simulink model "ADIA"  (R2018b)
settings: Solver=FixedStepDiscrete  StartTime=0.0  StopTime=10.0  FixedStep=0.02  RelTol=1e-3
undefined symbols (not defined in the file or in its folder): ACC_State_Active, ACC_State_BrakeOnly, ACC_State_Suspended, ACC_State_WaitingRise, ADAS_AEBBrakingProg, ADAS_DeclControlReq, ADAS_DriveOff, ADAS_ESCHoldReq_NotHold, ADASDecType_ACC, ADASDecType_AEB, ADIA_ACC_Acceleration_OOR_DecCount_C, ADIA_ACC_Acceleration_OOR_Duration_C, ADIA_ACC_Acceleration_OOR_IncCount_C, ADIA_ACC_Acceleration_OOR_LLim_C, ADIA_ACC_Acceleration_OOR_ULim_C, ADIA_ACC_AccelTrqReq_MixedDia_ULim_C, ADIA_ACC_AccelTrqReq_ULim_C, ADIA_ACC_Deceleration_Mixed_ULim_C, ADIA_ACC_Deceleration_OOR_DecCount_C, ADIA_ACC_Deceleration_OOR_Duration_C, ADIA_ACC_Deceleration_OOR_IncCount_C, ADIA_ACC_Deceleration_OOR_LLim_C, ADIA_ACC_Deceleration_OOR_ULim_C, ADIA_ACC_DriveOff_Distance_C, ADIA_ACC_DriveOff_TimeLim_C, ADIA_ACC_ReqMixed_DecCount_C, ADIA_ACC_ReqMixed_Duration_C, ADIA_ACC_ReqMixed_IncCount_C, ADIA_AccPedalRaw_MaxLim_C, ADIA_AccPedalRaw_MinLim_C, ADIA_ADAS_HoldDecReq_Set_C, ADIA_ADAS_HoldRConfirm_TimeLim_C, ADIA_ADAS_HoldVehSpd_Lim_C, ADIA_AEB_VehSpdDec_LLim_C, ADIA_AEB_VehSpdDec_ULim_C, ADIA_ASWFault_OvrdEn_C, ADIA_ASWFault_OvrdValue_C, ADIA_BatteryOutOfRange_DecCount_C, ADIA_BatteryOutOfRange_Duration_C, ADIA_BatteryOutOfRange_IncCount_C, ADIA_BattVolt_MaxLim_C, ADIA_BattVolt_MinLim_C, ADIA_BCM3_33C_InvBrkLight_DecCount_C, ADIA_BCM3_33C_InvBrkLight_Duration_C, ADIA_BCM3_33C_InvBrkLight_IncCount_C, ADIA_BCM_BattVolt_OvrdEn_C, ADIA_BCM_BattVolt_OvrdVal_C, ADIA_BCM_BrakeLampStaus_OvrdEn_C, ADIA_BCM_BrakeLampStaus_OvrdVal_C, ADIA_BCM_CHMSLStaus_OvrdEn_C, ADIA_BCM_CHMSLStaus_OvrdVal_C, ADIA_BCM_LeftTurnSwSt_OvrdEn_C, ADIA_BCM_LeftTurnSwSt_OvrdVal_C, ADIA_BCM_RightTurnSwSt_OvrdEn_C, ADIA_BCM_RightTurnSwSt_OvrdVal_C, ADIA_BCM_TurnSwFailure_DecCount_C, ADIA_BCM_TurnSwFailure_Duration_C, ADIA_BCM_TurnSwFailure_IncCount_C, ADIA_BSWFault_Ignore_C, ADIA_BSWFault_OvrdEn_C ... (+281)
libraries: simulink x208
(part 1 of 10)
settings Model: Creator=ZWG  LastModifiedBy=xiaoyang
settings OptimizationCC: DefaultParameterBehavior=Inlined  EnhancedBackFolding=on  PassReuseOutputArgsAs=Individual arguments  ZeroExternalMemoryAtStartup=off  ZeroInternalMemoryAtStartup=off  OptimizeBlockOrder=speed  DifferentSizesBufferReuse=on  OptimizationCustomize=off
settings DebuggingCC: ParameterTunabilityLossMsg=error
settings SFSimCC: MATLABDynamicMemAlloc=off
settings RTWCC: SystemTargetFile=autosar.tlc  GenCodeOnly=on  TemplateMakefile=ert_default_tmf  Description=AUTOSAR  GenerateReport=on  IncludeHyperlinkInReport=on  LaunchReport=on  GenerateTraceInfo=on  GenerateTraceReport=on  GenerateTraceReportSl=on  GenerateTraceReportSf=on  GenerateTraceReportEml=on
settings CodeAppCC: ForceParamTrailComments=on  IgnoreCustomStorageClasses=off  OperatorAnnotations=on  SimulinkDataObjDesc=on  SFDataObjDesc=on  InsertBlockDesc=on
settings STFCustomTargetCC: TargetLangStandard=C99 (ISO)  MultiwordLength=256  ParMdlRefBuildCompliant=on  CompOptLevelCompliant=on  IncludeMdlTerminateFcn=off  CombineOutputUpdateFcns=on  SuppressErrorStatus=on  ERTCustomFileBanners=on  SupportNonFinite=off  SupportComplex=off  SupportContinuousTime=off  SupportNonInlinedSFcns=off  RemoveResetFunc=on  MATLABClassNameForMDSCustomization=Simulink.SoftwareTarget.ERTCustomization  AutosarCompliant=on  UseToolchainInfoCompliant=on  LookupTableObjectStructAxisOrder=2,1,3,4,...  LUTObjectStructOrderEvenSpacing=Size,Table,Breakpoints  SystemTargetFile=autosar.tlc
settings ERTTargetCC: TargetLangStandard=C99 (ISO)  ConcurrentExecutionCompliant=off  IncludeMdlTerminateFcn=off  SuppressErrorStatus=on  SupportNonFinite=off  SupportComplex=off  ModelStepFunctionPrototypeControlCompliant=off  CPPClassGenCompliant=off  AutosarCompliant=on  LookupTableObjectStructAxisOrder=2,1,3,4,...  LUTObjectStructOrderEvenSpacing=Size,Table,Breakpoints  GenerateASAP2=on  InlinedParameterPlacement=NonHierarchical  ERTCustomFileTemplate=example_file_process.tlc

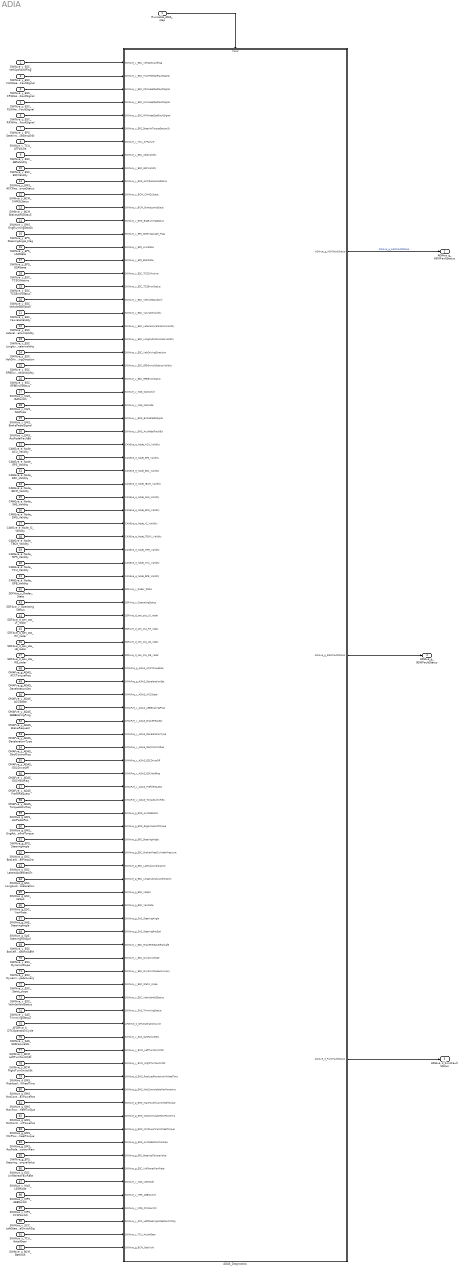
== system ADIA ==
  Runnable_ADIA_step : Inport  SampleTime=0.02  OutputFunctionCall=on
  SWINve_y_ESC_VehSpdValidFlag : Inport  Port=2  OutDataTypeStr=uint8
  SWINve_y_ESC_FLWHeelSpdFaultSignal : Inport  Port=3  OutDataTypeStr=uint8
  SWINve_y_ESC_FRWHeelSpdFaultSignal : Inport  Port=4  OutDataTypeStr=uint8
  SWINve_y_ESC_RLWHeelSpdFaultSignal : Inport  Port=5  OutDataTypeStr=uint8
  SWINve_y_ESC_RRWHeelSpdFaultSignal : Inport  Port=6  OutDataTypeStr=uint8
  SWINve_y_EPS_SteerintTorqueSensorSt : Inport  Port=7  OutDataTypeStr=uint8
  SWINve_y_TCU_ATFailure : Inport  Port=8  OutDataTypeStr=uint8
  SWINve_y_ESC_ABSValidity : Inport  Port=9  OutDataTypeStr=uint8
  SWINve_y_ESC_ESCValidity : Inport  Port=10  OutDataTypeStr=uint8
  SWINve_y_EMS_ACCResponseStatus : Inport  Port=11  OutDataTypeStr=uint8
  SWINve_y_BCM_CHMSLStaus : Inport  Port=12  OutDataTypeStr=uint8
  SWINve_y_BCM_BrakeLampStaus : Inport  Port=13  OutDataTypeStr=uint8
  SWINve_y_EMS_EngRunningStatus : Inport  Port=14  OutDataTypeStr=uint8
  SWINve_y_EPS_SteeringAngle_Flag : Inport  Port=15  OutDataTypeStr=uint8
  SWINve_y_EPS_LKAState : Inport  Port=16  OutDataTypeStr=uint8
  SWINve_y_EPS_ESAState : Inport  Port=17  OutDataTypeStr=uint8
  SWINve_y_ESC_TCSCtlActive : Inport  Port=18  OutDataTypeStr=uint8
  SWINve_y_ESC_TCSErrorStatus : Inport  Port=19  OutDataTypeStr=uint8
  SWINve_y_ESC_VehicleStandstill : Inport  Port=20  OutDataTypeStr=uint8
  SWINve_y_ESC_YawrateValidity : Inport  Port=21  OutDataTypeStr=uint8
  SWINve_y_ESC_LateralAccelarationValidity : Inport  Port=22  OutDataTypeStr=uint8
  SWINve_y_ESC_LongitudinalAccelervalidity : Inport  Port=23  OutDataTypeStr=uint8
  SWINve_y_ESC_VehDrivingDirection : Inport  Port=24  OutDataTypeStr=uint8
  SWINve_y_ESC_EPBSwitchStaticsValidity : Inport  Port=25  OutDataTypeStr=uint8
  SWINve_y_ESC_EPBErrorStatus : Inport  Port=26  OutDataTypeStr=uint8
  SWINve_y_Mp5_ISASwitch : Inport  Port=27  OutDataTypeStr=uint8
  SWINve_y_Mp5_ISAMode : Inport  Port=28  OutDataTypeStr=uint8
  SWINve_y_EMS_BrakePedalSignal : Inport  Port=29  OutDataTypeStr=uint8
  SWINve_y_EMS_AccPedalFaultBit : Inport  Port=30  OutDataTypeStr=uint8
  CANEve_e_Node_ACU_Validity : Inport  Port=31  OutDataTypeStr=Enum: SPARte_e_Validity  PortDimensions=1
  CANEve_e_Node_EPS_Validity : Inport  Port=32  OutDataTypeStr=Enum: SPARte_e_Validity  PortDimensions=1
  CANEve_e_Node_ESC_Validity : Inport  Port=33  OutDataTypeStr=Enum: SPARte_e_Validity  PortDimensions=1
  CANEve_e_Node_IBCM_Validity : Inport  Port=34  OutDataTypeStr=Enum: SPARte_e_Validity  PortDimensions=1
  CANEve_e_Node_SAS_Validity : Inport  Port=35  OutDataTypeStr=Enum: SPARte_e_Validity  PortDimensions=1
  CANEve_e_Node_EMS_Validity : Inport  Port=36  OutDataTypeStr=Enum: SPARte_e_Validity  PortDimensions=1
  CANEve_e_Node_IC_Validity : Inport  Port=37  OutDataTypeStr=Enum: SPARte_e_Validity  PortDimensions=1
  CANEve_e_Node_TBOX_Validity : Inport  Port=38  OutDataTypeStr=Enum: SPARte_e_Validity  PortDimensions=1
  CANEve_e_Node_MP5_Validity : Inport  Port=39  OutDataTypeStr=Enum: SPARte_e_Validity  PortDimensions=1
  CANEve_e_Node_TCU_Validity : Inport  Port=40  OutDataTypeStr=Enum: SPARte_e_Validity  PortDimensions=1
  CANEve_e_Node_EPB_Validity : Inport  Port=41  OutDataTypeStr=Enum: SPARte_e_Validity  PortDimensions=1
  SDFAve_y_Radar_State : Inport  Port=42  OutDataTypeStr=UInt8
  SDFAve_y_OperatingStatus : Inport  Port=43  OutDataTypeStr=UInt8
  SDFAve_d_sen_sta_LF_radar : Inport  Port=44  OutDataTypeStr=UInt16
  SDFAve_d_sen_sta_RF_radar : Inport  Port=45  OutDataTypeStr=UInt16
  SDFAve_d_sen_sta_LB_radar : Inport  Port=46  OutDataTypeStr=UInt16
  SDFAve_d_sen_sta_RB_radar : Inport  Port=47  OutDataTypeStr=UInt16
  OMAPve_g_ADAS_ACCTorqueReq : Inport  Port=48  OutDataTypeStr=T_M_Nm_Float32  PortDimensions=1
  OMAPve_g_ADAS_DecelerationSet : Inport  Port=49  OutDataTypeStr=T_M_Nm_Float32  PortDimensions=1
  OMAPve_y_ADAS_ACCState : Inport  Port=50  OutDataTypeStr=UInt8  PortDimensions=1
  OMAPve_y_ADAS_AEBBrakingProg : Inport  Port=51  OutDataTypeStr=UInt8  PortDimensions=1
  OMAPve_y_ADAS_BrakeRequest : Inport  Port=52  OutDataTypeStr=UInt8  PortDimensions=1
  OMAPve_y_ADAS_DecelerationType : Inport  Port=53  OutDataTypeStr=UInt8  PortDimensions=1
  OMAPve_y_ADAS_DeclControlReq : Inport  Port=54  OutDataTypeStr=UInt8  PortDimensions=1
  OMAPve_y_ADAS_ESCDriveOff : Inport  Port=55  OutDataTypeStr=UInt8  PortDimensions=1
  OMAPve_y_ADAS_ESCHoldReq : Inport  Port=56  OutDataTypeStr=UInt8  PortDimensions=1
  OMAPve_y_ADAS_PrefillRequest : Inport  Port=57  OutDataTypeStr=UInt8  PortDimensions=1
  OMAPve_y_ADAS_TorqueActivReq : Inport  Port=58  OutDataTypeStr=UInt8  PortDimensions=1
  SWINve_g_EMS_AccPedalPos : Inport  Port=59  OutDataTypeStr=single  PortDimensions=1
  SWINve_g_EMS_EngActualIndTorque : Inport  Port=60  OutDataTypeStr=single  PortDimensions=1
  SWINve_g_EPS_SteeringAngle : Inport  Port=61  OutDataTypeStr=single  PortDimensions=1
  SWINve_g_ESC_BrakeWheelCylinderPressure : Inport  Port=62  OutDataTypeStr=single  PortDimensions=1
  SWINve_g_ESC_LateralAccelaration : Inport  Port=63  OutDataTypeStr=single  PortDimensions=1
  SWINve_g_ESC_LongitudinalAcceleration : Inport  Port=64  OutDataTypeStr=single  PortDimensions=1
  SWINve_g_ESC_VeSpd : Inport  Port=65  OutDataTypeStr=single  PortDimensions=1
  SWINve_g_ESC_YawRate : Inport  Port=66  OutDataTypeStr=single  PortDimensions=1
  SWINve_g_SAS_SteeringAngle : Inport  Port=67  OutDataTypeStr=T_M_Nm_Float32  PortDimensions=1
  SWINve_g_SAS_SteeringRotSpd : Inport  Port=68  OutDataTypeStr=single  PortDimensions=1
  SWINve_y_ESC_BrakeReleasedFailsafe : Inport  Port=69  OutDataTypeStr=uint8  PortDimensions=1
  SWINve_y_ESC_DynamicSlope : Inport  Port=70  OutDataTypeStr=int8  PortDimensions=1
  SWINve_y_ESC_DynamicSlopeAccuracy : Inport  Port=71  OutDataTypeStr=uint8  PortDimensions=1
  SWINve_y_ESC_Static_slope : Inport  Port=72  OutDataTypeStr=int8  PortDimensions=1
  SWINve_y_ESC_VehicleHoldStatus : Inport  Port=73  OutDataTypeStr=uint8  PortDimensions=1
  SWINve_y_SAS_TrimmingStatus : Inport  Port=74  OutDataTypeStr=uint8  PortDimensions=1
  AFDMve_b_DTCOperationCycle : Inport  Port=75  OutDataTypeStr=T_BOOLEAN  PortDimensions=1
  SWINve_y_SAS_SASFailureSts : Inport  Port=76  OutDataTypeStr=uint8
  SWINve_y_BCM_LeftTurnSwitchSt : Inport  Port=77  OutDataTypeStr=uint8
  SWINve_y_BCM_RightTurnSwitchSt : Inport  Port=78  OutDataTypeStr=uint8
  SWINve_d_EMS_RealizedPowertrainWheelTorq : Inport  Port=79  OutDataTypeStr=int16
  SWINve_g_EMS_NotControlableMaxPowertra : Inport  Port=80  OutDataTypeStr=single
  SWINve_g_EMS_MaxPowertrainWheelTorque : Inport  Port=81  OutDataTypeStr=single
  SWINve_g_EMS_NotControlableMinPowertra : Inport  Port=82  OutDataTypeStr=single
  SWINve_g_EMS_MinPowertrainWheelTorque : Inport  Port=83  OutDataTypeStr=single
  SWINve_g_EMS_AccPedalPositionRaw : Inport  Port=84  OutDataTypeStr=single
  SWINve_g_EPS_SteeringTorqueValue : Inport  Port=85  OutDataTypeStr=single
  SWINve_g_ESC_UnfilteredYawRate : Inport  Port=86  OutDataTypeStr=single  PortDimensions=1
  SWINve_y_Mp5_LSSMode : Inport  Port=87  OutDataTypeStr=uint8  PortDimensions=1
  SWINve_y_MP5_AEBSwitch : Inport  Port=88  OutDataTypeStr=uint8  PortDimensions=1
  SWINve_y_MP5_FCWSwitch : Inport  Port=89  OutDataTypeStr=uint8  PortDimensions=1
  SWINve_y_SCC_LeftSteeringWheelSwitchSig : Inport  Port=90  OutDataTypeStr=uint8  PortDimensions=1
  SWINve_y_TCU_ActialGear : Inport  Port=91  OutDataTypeStr=uint8  PortDimensions=1
  SWINve_g_BCM_BattVolt : Inport  Port=92  OutDataTypeStr=single  PortDimensions=1
  ADAS_Diagnostics : Subsystem
  ADIAve_g_ASWFaultStatus : Outport  OutDataTypeStr=UInt32
  ADIAve_g_BSWFaultStatus : Outport  Port=2  OutDataTypeStr=UInt32
  ADIAve_d_FuncFaultStatus : Outport  Port=3  OutDataTypeStr=uint16
  wires:
  SDFAve_d_sen_sta_RB_radar/1 -> ADAS_Diagnostics/46(SDFAve_d_sen_sta_RB_radar)
  SWINve_y_ESC_RRWHeelSpdFaultSignal/1 -> ADAS_Diagnostics/5(SWINve_y_ESC_RRWHeelSpdFaultSignal)
  SDFAve_d_sen_sta_LB_radar/1 -> ADAS_Diagnostics/45(SDFAve_d_sen_sta_LB_radar)
  SDFAve_d_sen_sta_RF_radar/1 -> ADAS_Diagnostics/44(SDFAve_d_sen_sta_RF_radar)
  SWINve_y_EMS_EngRunningStatus/1 -> ADAS_Diagnostics/13(SWINve_y_EMS_EngRunningStatus)
  CANEve_e_Node_IBCM_Validity/1 -> ADAS_Diagnostics/33(CANEve_e_Node_IBCM_Validity)
  SDFAve_d_sen_sta_LF_radar/1 -> ADAS_Diagnostics/43(SDFAve_d_sen_sta_LF_radar)
  SDFAve_y_OperatingStatus/1 -> ADAS_Diagnostics/42(SDFAve_y_OperatingStatus)
  SWINve_y_ESC_ABSValidity/1 -> ADAS_Diagnostics/8(SWINve_y_ESC_ABSValidity)
  CANEve_e_Node_MP5_Validity/1 -> ADAS_Diagnostics/38(CANEve_e_Node_MP5_Validity)
  SWINve_y_BCM_CHMSLStaus/1 -> ADAS_Diagnostics/11(SWINve_y_BCM_CHMSLStaus)
  SDFAve_y_Radar_State/1 -> ADAS_Diagnostics/41(SDFAve_y_Radar_State)
  CANEve_e_Node_ESC_Validity/1 -> ADAS_Diagnostics/32(CANEve_e_Node_ESC_Validity)
  CANEve_e_Node_TBOX_Validity/1 -> ADAS_Diagnostics/37(CANEve_e_Node_TBOX_Validity)
  SWINve_y_EPS_SteerintTorqueSensorSt/1 -> ADAS_Diagnostics/6(SWINve_y_EPS_SteerintTorqueSensorSt)
  SWINve_y_ESC_LongitudinalAccelervalidity/1 -> ADAS_Diagnostics/22(SWINve_y_ESC_LongitudinalAccelervalidity)
  CANEve_e_Node_ACU_Validity/1 -> ADAS_Diagnostics/30(CANEve_e_Node_ACU_Validity)
  SWINve_y_ESC_RLWHeelSpdFaultSignal/1 -> ADAS_Diagnostics/4(SWINve_y_ESC_RLWHeelSpdFaultSignal)
  CANEve_e_Node_EMS_Validity/1 -> ADAS_Diagnostics/35(CANEve_e_Node_EMS_Validity)
  CANEve_e_Node_EPS_Validity/1 -> ADAS_Diagnostics/31(CANEve_e_Node_EPS_Validity)
  CANEve_e_Node_IC_Validity/1 -> ADAS_Diagnostics/36(CANEve_e_Node_IC_Validity)
  SWINve_y_ESC_YawrateValidity/1 -> ADAS_Diagnostics/20(SWINve_y_ESC_YawrateValidity)
  SWINve_y_Mp5_ISASwitch/1 -> ADAS_Diagnostics/26(SWINve_y_Mp5_ISASwitch)
  SWINve_y_ESC_EPBSwitchStaticsValidity/1 -> ADAS_Diagnostics/24(SWINve_y_ESC_EPBSwitchStaticsValidity)
  SWINve_y_EPS_ESAState/1 -> ADAS_Diagnostics/16(SWINve_y_EPS_ESAState)
  CANEve_e_Node_SAS_Validity/1 -> ADAS_Diagnostics/34(CANEve_e_Node_SAS_Validity)
  SWINve_y_BCM_BrakeLampStaus/1 -> ADAS_Diagnostics/12(SWINve_y_BCM_BrakeLampStaus)
  Runnable_ADIA_step/1 -> ADAS_Diagnostics/Trigger
  SWINve_y_EMS_ACCResponseStatus/1 -> ADAS_Diagnostics/10(SWINve_y_EMS_ACCResponseStatus)
  SWINve_y_ESC_EPBErrorStatus/1 -> ADAS_Diagnostics/25(SWINve_y_ESC_EPBErrorStatus)
  SWINve_y_EPS_SteeringAngle_Flag/1 -> ADAS_Diagnostics/14(SWINve_y_EPS_SteeringAngle_Flag)
  SWINve_y_ESC_FRWHeelSpdFaultSignal/1 -> ADAS_Diagnostics/3(SWINve_y_ESC_FRWHeelSpdFaultSignal)
  ADAS_Diagnostics/2(ADIAve_g_BSWFaultStatus) -> ADIAve_g_BSWFaultStatus/1
  SWINve_y_ESC_ESCValidity/1 -> ADAS_Diagnostics/9(SWINve_y_ESC_ESCValidity)
  SWINve_y_TCU_ATFailure/1 -> ADAS_Diagnostics/7(SWINve_y_TCU_ATFailure)
  SWINve_y_ESC_FLWHeelSpdFaultSignal/1 -> ADAS_Diagnostics/2(SWINve_y_ESC_FLWHeelSpdFaultSignal)
  SWINve_y_EPS_LKAState/1 -> ADAS_Diagnostics/15(SWINve_y_EPS_LKAState)
  ADAS_Diagnostics/1(ADIAve_g_ASWFaultStatus) -> ADIAve_g_ASWFaultStatus/1  "ADIAve_g_ASWFaultStatus"
  AFDMve_b_DTCOperationCycle/1 -> ADAS_Diagnostics/74(AFDMve_b_DTCOperationCycle)
  SWINve_y_ESC_VehicleStandstill/1 -> ADAS_Diagnostics/19(SWINve_y_ESC_VehicleStandstill)
  CANEve_e_Node_TCU_Validity/1 -> ADAS_Diagnostics/39(CANEve_e_Node_TCU_Validity)
  CANEve_e_Node_EPB_Validity/1 -> ADAS_Diagnostics/40(CANEve_e_Node_EPB_Validity)
  SWINve_y_ESC_LateralAccelarationValidity/1 -> ADAS_Diagnostics/21(SWINve_y_ESC_LateralAccelarationValidity)
  SWINve_y_ESC_TCSCtlActive/1 -> ADAS_Diagnostics/17(SWINve_y_ESC_TCSCtlActive)
  SWINve_y_EMS_AccPedalFaultBit/1 -> ADAS_Diagnostics/29(SWINve_y_EMS_AccPedalFaultBit)
  SWINve_y_ESC_TCSErrorStatus/1 -> ADAS_Diagnostics/18(SWINve_y_ESC_TCSErrorStatus)
  SWINve_y_ESC_VehDrivingDirection/1 -> ADAS_Diagnostics/23(SWINve_y_ESC_VehDrivingDirection)
  SWINve_y_ESC_VehSpdValidFlag/1 -> ADAS_Diagnostics/1(SWINve_y_ESC_VehSpdValidFlag)
  SWINve_y_Mp5_ISAMode/1 -> ADAS_Diagnostics/27(SWINve_y_Mp5_ISAMode)
  SWINve_y_EMS_BrakePedalSignal/1 -> ADAS_Diagnostics/28(SWINve_y_EMS_BrakePedalSignal)
  SWINve_y_SAS_TrimmingStatus/1 -> ADAS_Diagnostics/73(SWINve_y_SAS_TrimmingStatus)
  SWINve_y_ESC_VehicleHoldStatus/1 -> ADAS_Diagnostics/72(SWINve_y_ESC_VehicleHoldStatus)
  SWINve_y_ESC_Static_slope/1 -> ADAS_Diagnostics/71(SWINve_y_ESC_Static_slope)
  SWINve_y_ESC_DynamicSlopeAccuracy/1 -> ADAS_Diagnostics/70(SWINve_y_ESC_DynamicSlopeAccuracy)
  SWINve_y_ESC_DynamicSlope/1 -> ADAS_Diagnostics/69(SWINve_y_ESC_DynamicSlope)
  SWINve_y_ESC_BrakeReleasedFailsafe/1 -> ADAS_Diagnostics/68(SWINve_y_ESC_BrakeReleasedFailsafe)
  SWINve_g_SAS_SteeringRotSpd/1 -> ADAS_Diagnostics/67(SWINve_g_SAS_SteeringRotSpd)
  SWINve_g_SAS_SteeringAngle/1 -> ADAS_Diagnostics/66(SWINve_g_SAS_SteeringAngle)
  SWINve_g_ESC_YawRate/1 -> ADAS_Diagnostics/65(SWINve_g_ESC_YawRate)
  SWINve_g_ESC_VeSpd/1 -> ADAS_Diagnostics/64(SWINve_g_ESC_VeSpd)
  SWINve_g_ESC_LongitudinalAcceleration/1 -> ADAS_Diagnostics/63(SWINve_g_ESC_LongitudinalAcceleration)
  SWINve_g_ESC_LateralAccelaration/1 -> ADAS_Diagnostics/62(SWINve_g_ESC_LateralAccelaration)
  SWINve_g_ESC_BrakeWheelCylinderPressure/1 -> ADAS_Diagnostics/61(SWINve_g_ESC_BrakeWheelCylinderPressure)
  SWINve_g_EPS_SteeringAngle/1 -> ADAS_Diagnostics/60(SWINve_g_EPS_SteeringAngle)
  SWINve_g_EMS_EngActualIndTorque/1 -> ADAS_Diagnostics/59(SWINve_g_EMS_EngActualIndTorque)
  SWINve_g_EMS_AccPedalPos/1 -> ADAS_Diagnostics/58(SWINve_g_EMS_AccPedalPos)
  OMAPve_y_ADAS_TorqueActivReq/1 -> ADAS_Diagnostics/57(OMAPve_y_ADAS_TorqueActivReq)
  OMAPve_y_ADAS_PrefillRequest/1 -> ADAS_Diagnostics/56(OMAPve_y_ADAS_PrefillRequest)
  OMAPve_y_ADAS_ESCHoldReq/1 -> ADAS_Diagnostics/55(OMAPve_y_ADAS_ESCHoldReq)
  OMAPve_y_ADAS_ESCDriveOff/1 -> ADAS_Diagnostics/54(OMAPve_y_ADAS_ESCDriveOff)
  OMAPve_y_ADAS_DeclControlReq/1 -> ADAS_Diagnostics/53(OMAPve_y_ADAS_DeclControlReq)
  OMAPve_y_ADAS_DecelerationType/1 -> ADAS_Diagnostics/52(OMAPve_y_ADAS_DecelerationType)
  OMAPve_y_ADAS_BrakeRequest/1 -> ADAS_Diagnostics/51(OMAPve_y_ADAS_BrakeRequest)
  OMAPve_y_ADAS_AEBBrakingProg/1 -> ADAS_Diagnostics/50(OMAPve_y_ADAS_AEBBrakingProg)
  OMAPve_y_ADAS_ACCState/1 -> ADAS_Diagnostics/49(OMAPve_y_ADAS_ACCState)
  OMAPve_g_ADAS_DecelerationSet/1 -> ADAS_Diagnostics/48(OMAPve_g_ADAS_DecelerationSet)
  OMAPve_g_ADAS_ACCTorqueReq/1 -> ADAS_Diagnostics/47(OMAPve_g_ADAS_ACCTorqueReq)
  SWINve_y_SAS_SASFailureSts/1 -> ADAS_Diagnostics/75(SWINve_y_SAS_SASFailureSts)
  SWINve_y_BCM_LeftTurnSwitchSt/1 -> ADAS_Diagnostics/76(SWINve_y_BCM_LeftTurnSwitchSt)
  SWINve_y_BCM_RightTurnSwitchSt/1 -> ADAS_Diagnostics/77(SWINve_y_BCM_RightTurnSwitchSt)
  SWINve_d_EMS_RealizedPowertrainWheelTorq/1 -> ADAS_Diagnostics/78(SWINve_d_EMS_RealizedPowertrainWheelTorq)
  SWINve_g_EMS_NotControlableMaxPowertra/1 -> ADAS_Diagnostics/79(SWINve_g_EMS_NotControlableMaxPowertra)
  SWINve_g_EMS_MaxPowertrainWheelTorque/1 -> ADAS_Diagnostics/80(SWINve_g_EMS_MaxPowertrainWheelTorque)
  SWINve_g_EMS_NotControlableMinPowertra/1 -> ADAS_Diagnostics/81(SWINve_g_EMS_NotControlableMinPowertra)
  SWINve_g_EMS_MinPowertrainWheelTorque/1 -> ADAS_Diagnostics/82(SWINve_g_EMS_MinPowertrainWheelTorque)
  SWINve_g_EMS_AccPedalPositionRaw/1 -> ADAS_Diagnostics/83(SWINve_g_EMS_AccPedalPositionRaw)
  SWINve_g_EPS_SteeringTorqueValue/1 -> ADAS_Diagnostics/84(SWINve_g_EPS_SteeringTorqueValue)
  SWINve_g_ESC_UnfilteredYawRate/1 -> ADAS_Diagnostics/85(SWINve_g_ESC_UnfilteredYawRate)
  SWINve_y_MP5_AEBSwitch/1 -> ADAS_Diagnostics/87(SWINve_y_MP5_AEBSwitch)
  SWINve_y_Mp5_LSSMode/1 -> ADAS_Diagnostics/86(SWINve_y_Mp5_LSSMode)
  SWINve_y_MP5_FCWSwitch/1 -> ADAS_Diagnostics/88(SWINve_y_MP5_FCWSwitch)
  SWINve_y_TCU_ActialGear/1 -> ADAS_Diagnostics/90(SWINve_y_TCU_ActialGear)
  SWINve_y_SCC_LeftSteeringWheelSwitchSig/1 -> ADAS_Diagnostics/89(SWINve_y_SCC_LeftSteeringWheelSwitchSig)
  SWINve_g_BCM_BattVolt/1 -> ADAS_Diagnostics/91(SWINve_g_BCM_BattVolt)
  ADAS_Diagnostics/3(ADIAve_d_FuncFaultStatus) -> ADIAve_d_FuncFaultStatus/1

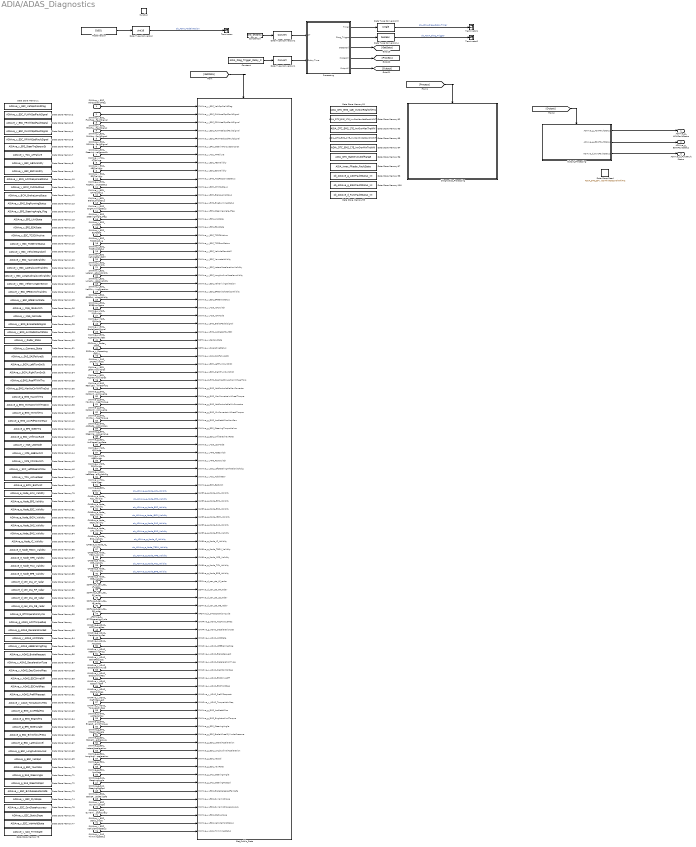
== system ADIA/ADAS_Diagnostics ==
  SWINve_y_ESC_VehSpdValidFlag : Inport
  SWINve_y_ESC_FLWHeelSpdFaultSignal : Inport  Port=2
  SWINve_y_ESC_FRWHeelSpdFaultSignal : Inport  Port=3
  SWINve_y_ESC_RLWHeelSpdFaultSignal : Inport  Port=4
  SWINve_y_ESC_RRWHeelSpdFaultSignal : Inport  Port=5
  SWINve_y_EPS_SteerintTorqueSensorSt : Inport  Port=6
  SWINve_y_TCU_ATFailure : Inport  Port=7
  SWINve_y_ESC_ABSValidity : Inport  Port=8
  SWINve_y_ESC_ESCValidity : Inport  Port=9
  SWINve_y_EMS_ACCResponseStatus : Inport  Port=10
  SWINve_y_BCM_CHMSLStaus : Inport  Port=11
  SWINve_y_BCM_BrakeLampStaus : Inport  Port=12
  SWINve_y_EMS_EngRunningStatus : Inport  Port=13
  SWINve_y_EPS_SteeringAngle_Flag : Inport  Port=14
  SWINve_y_EPS_LKAState : Inport  Port=15
  SWINve_y_EPS_ESAState : Inport  Port=16
  SWINve_y_ESC_TCSCtlActive : Inport  Port=17
  SWINve_y_ESC_TCSErrorStatus : Inport  Port=18
  SWINve_y_ESC_VehicleStandstill : Inport  Port=19
  SWINve_y_ESC_YawrateValidity : Inport  Port=20
  SWINve_y_ESC_LateralAccelarationValidity : Inport  Port=21
  SWINve_y_ESC_LongitudinalAccelervalidity : Inport  Port=22
  SWINve_y_ESC_VehDrivingDirection : Inport  Port=23
  SWINve_y_ESC_EPBSwitchStaticsValidity : Inport  Port=24
  SWINve_y_ESC_EPBErrorStatus : Inport  Port=25
  SWINve_y_Mp5_ISASwitch : Inport  Port=26
  SWINve_y_Mp5_ISAMode : Inport  Port=27
  SWINve_y_EMS_BrakePedalSignal : Inport  Port=28
  SWINve_y_EMS_AccPedalFaultBit : Inport  Port=29
  CANEve_e_Node_ACU_Validity : Inport  Port=30  PortDimensions=1
  CANEve_e_Node_EPS_Validity : Inport  Port=31  PortDimensions=1
  CANEve_e_Node_ESC_Validity : Inport  Port=32  PortDimensions=1
  CANEve_e_Node_IBCM_Validity : Inport  Port=33  PortDimensions=1
  CANEve_e_Node_SAS_Validity : Inport  Port=34  PortDimensions=1
  CANEve_e_Node_EMS_Validity : Inport  Port=35  PortDimensions=1
  CANEve_e_Node_IC_Validity : Inport  Port=36  PortDimensions=1
  CANEve_e_Node_TBOX_Validity : Inport  Port=37  PortDimensions=1
  CANEve_e_Node_MP5_Validity : Inport  Port=38  PortDimensions=1
  CANEve_e_Node_TCU_Validity : Inport  Port=39  PortDimensions=1
  CANEve_e_Node_EPB_Validity : Inport  Port=40  PortDimensions=1
  SDFAve_y_Radar_State : Inport  Port=41
  SDFAve_y_OperatingStatus : Inport  Port=42
  SDFAve_d_sen_sta_LF_radar : Inport  Port=43
  SDFAve_d_sen_sta_RF_radar : Inport  Port=44
  SDFAve_d_sen_sta_LB_radar : Inport  Port=45
  SDFAve_d_sen_sta_RB_radar : Inport  Port=46
  OMAPve_g_ADAS_ACCTorqueReq : Inport  Port=47  OutDataTypeStr=T_M_Nm_Float32  PortDimensions=1
  OMAPve_g_ADAS_DecelerationSet : Inport  Port=48  OutDataTypeStr=T_M_Nm_Float32  PortDimensions=1
  OMAPve_y_ADAS_ACCState : Inport  Port=49  OutDataTypeStr=UInt8  PortDimensions=1
  OMAPve_y_ADAS_AEBBrakingProg : Inport  Port=50  OutDataTypeStr=UInt8  PortDimensions=1
  OMAPve_y_ADAS_BrakeRequest : Inport  Port=51  OutDataTypeStr=UInt8  PortDimensions=1
  OMAPve_y_ADAS_DecelerationType : Inport  Port=52  OutDataTypeStr=UInt8  PortDimensions=1
  OMAPve_y_ADAS_DeclControlReq : Inport  Port=53  OutDataTypeStr=UInt8  PortDimensions=1
  OMAPve_y_ADAS_ESCDriveOff : Inport  Port=54  OutDataTypeStr=UInt8  PortDimensions=1
  OMAPve_y_ADAS_ESCHoldReq : Inport  Port=55  OutDataTypeStr=UInt8  PortDimensions=1
  OMAPve_y_ADAS_PrefillRequest : Inport  Port=56  OutDataTypeStr=UInt8  PortDimensions=1
  OMAPve_y_ADAS_TorqueActivReq : Inport  Port=57  OutDataTypeStr=UInt8  PortDimensions=1
  SWINve_g_EMS_AccPedalPos : Inport  Port=58  OutDataTypeStr=single  PortDimensions=1
  SWINve_g_EMS_EngActualIndTorque : Inport  Port=59  OutDataTypeStr=single  PortDimensions=1
  SWINve_g_EPS_SteeringAngle : Inport  Port=60  OutDataTypeStr=single  PortDimensions=1
  SWINve_g_ESC_BrakeWheelCylinderPressure : Inport  Port=61  OutDataTypeStr=single  PortDimensions=1
  SWINve_g_ESC_LateralAccelaration : Inport  Port=62  OutDataTypeStr=single  PortDimensions=1
  SWINve_g_ESC_LongitudinalAcceleration : Inport  Port=63  OutDataTypeStr=single  PortDimensions=1
  SWINve_g_ESC_VeSpd : Inport  Port=64  OutDataTypeStr=single  PortDimensions=1
  SWINve_g_ESC_YawRate : Inport  Port=65  PortDimensions=1
  SWINve_g_SAS_SteeringAngle : Inport  Port=66  OutDataTypeStr=T_M_Nm_Float32  PortDimensions=1
  SWINve_g_SAS_SteeringRotSpd : Inport  Port=67  OutDataTypeStr=single  PortDimensions=1
  SWINve_y_ESC_BrakeReleasedFailsafe : Inport  Port=68  OutDataTypeStr=uint8  PortDimensions=1
  SWINve_y_ESC_DynamicSlope : Inport  Port=69  OutDataTypeStr=int8  PortDimensions=1
  SWINve_y_ESC_DynamicSlopeAccuracy : Inport  Port=70  OutDataTypeStr=uint8  PortDimensions=1
  SWINve_y_ESC_Static_slope : Inport  Port=71  OutDataTypeStr=int8  PortDimensions=1
  SWINve_y_ESC_VehicleHoldStatus : Inport  Port=72  OutDataTypeStr=uint8  PortDimensions=1
  SWINve_y_SAS_TrimmingStatus : Inport  Port=73  OutDataTypeStr=uint8  PortDimensions=1
  AFDMve_b_DTCOperationCycle : Inport  Port=74  OutDataTypeStr=T_BOOLEAN  PortDimensions=1
  SWINve_y_SAS_SASFailureSts : Inport  Port=75
  SWINve_y_BCM_LeftTurnSwitchSt : Inport  Port=76
  SWINve_y_BCM_RightTurnSwitchSt : Inport  Port=77
  SWINve_d_EMS_RealizedPowertrainWheelTorq : Inport  Port=78
  SWINve_g_EMS_NotControlableMaxPowertra : Inport  Port=79
  SWINve_g_EMS_MaxPowertrainWheelTorque : Inport  Port=80
  SWINve_g_EMS_NotControlableMinPowertra : Inport  Port=81
  SWINve_g_EMS_MinPowertrainWheelTorque : Inport  Port=82
  SWINve_g_EMS_AccPedalPositionRaw : Inport  Port=83
  SWINve_g_EPS_SteeringTorqueValue : Inport  Port=84
  SWINve_g_ESC_UnfilteredYawRate : Inport  Port=85  PortDimensions=1
  SWINve_y_Mp5_LSSMode : Inport  Port=86  OutDataTypeStr=uint8  PortDimensions=1
  SWINve_y_MP5_AEBSwitch : Inport  Port=87  OutDataTypeStr=uint8  PortDimensions=1
  SWINve_y_MP5_FCWSwitch : Inport  Port=88  OutDataTypeStr=uint8  PortDimensions=1
  SWINve_y_SCC_LeftSteeringWheelSwitchSig : Inport  Port=89  PortDimensions=1
  SWINve_y_TCU_ActialGear : Inport  Port=90  PortDimensions=1
  SWINve_g_BCM_BattVolt : Inport  Port=91  OutDataTypeStr=single  PortDimensions=1
  function : TriggerPort  TriggerType=function-call  VariantControl=Variant  SampleTimeType=periodic  SampleTime=-1
  Constant : Constant  Value=ADIA_Diag_Trigger_Delay_C  SampleTime=-1
  Constant10 : Constant  Value=SYS_dT20ms
  Data Store Memory : DataStoreMemory  DataStoreName=ADIAve_g_ADAS_ACCTorqueReq  ShowAdditionalParam=off  StateMustResolveToSignalObject=on
  Data Store Memory1 : DataStoreMemory  DataStoreName=ADIAve_y_ESC_VehSpdValidFlag  ShowAdditionalParam=off  StateMustResolveToSignalObject=on
  Data Store Memory10 : DataStoreMemory  DataStoreName=ADIAve_y_EMS_ACCResponseStatus  ShowAdditionalParam=off  StateMustResolveToSignalObject=on
  Data Store Memory100 : DataStoreMemory  DataStoreName=ob_ADIAve_g_BSWFaultStatus_ini  ShowAdditionalParam=off  StateMustResolveToSignalObject=on
  Data Store Memory11 : DataStoreMemory  DataStoreName=ADIAve_y_BCM_CHMSLStaus  ShowAdditionalParam=off  StateMustResolveToSignalObject=on
  Data Store Memory12 : DataStoreMemory  DataStoreName=ADIAve_y_BCM_BrakeLampStaus  ShowAdditionalParam=off  StateMustResolveToSignalObject=on
  Data Store Memory13 : DataStoreMemory  DataStoreName=ADIAve_y_EMS_EngRunningStatus  ShowAdditionalParam=off  StateMustResolveToSignalObject=on
  Data Store Memory14 : DataStoreMemory  DataStoreName=ADIAve_y_EPS_SteeringAngle_Flag  ShowAdditionalParam=off  StateMustResolveToSignalObject=on
  Data Store Memory15 : DataStoreMemory  DataStoreName=ADIAve_y_EPS_LKAState  ShowAdditionalParam=off  StateMustResolveToSignalObject=on
  Data Store Memory16 : DataStoreMemory  DataStoreName=ADIAve_y_EPS_ESAState  ShowAdditionalParam=off  StateMustResolveToSignalObject=on
  Data Store Memory17 : DataStoreMemory  DataStoreName=ADIAve_y_ESC_TCSCtlActive  ShowAdditionalParam=off  StateMustResolveToSignalObject=on
  Data Store Memory18 : DataStoreMemory  DataStoreName=ADIAve_y_ESC_TCSErrorStatus  ShowAdditionalParam=off  StateMustResolveToSignalObject=on
  Data Store Memory19 : DataStoreMemory  DataStoreName=ADIAve_y_ESC_VehicleStandstill  ShowAdditionalParam=off  StateMustResolveToSignalObject=on
  Data Store Memory2 : DataStoreMemory  DataStoreName=ADIAve_y_ESC_FLWhlSpdFaultSignal  ShowAdditionalParam=off  StateMustResolveToSignalObject=on
  Data Store Memory20 : DataStoreMemory  DataStoreName=ADIAve_y_ESC_YawrateValidity  ShowAdditionalParam=off  StateMustResolveToSignalObject=on
  Data Store Memory21 : DataStoreMemory  DataStoreName=ADIAve_y_ESC_LateralAccelValidity  ShowAdditionalParam=off  StateMustResolveToSignalObject=on
  Data Store Memory22 : DataStoreMemory  DataStoreName=ADIAve_y_ESC_LongitudinalAccelValidity  ShowAdditionalParam=off  StateMustResolveToSignalObject=on
  Data Store Memory23 : DataStoreMemory  DataStoreName=ADIAve_y_ESC_VehDrivingDirection  ShowAdditionalParam=off  StateMustResolveToSignalObject=on
  Data Store Memory24 : DataStoreMemory  DataStoreName=ADIAve_y_ESC_EPBSwitchValidity  ShowAdditionalParam=off  StateMustResolveToSignalObject=on
  Data Store Memory25 : DataStoreMemory  DataStoreName=ADIAve_y_ESC_EPBErrorState  ShowAdditionalParam=off  StateMustResolveToSignalObject=on
  Data Store Memory26 : DataStoreMemory  DataStoreName=ADIAve_y_Mp5_ISASwitch  ShowAdditionalParam=off  StateMustResolveToSignalObject=on
  Data Store Memory27 : DataStoreMemory  DataStoreName=ADIAve_y_Mp5_ISAMode  ShowAdditionalParam=off  StateMustResolveToSignalObject=on
  Data Store Memory28 : DataStoreMemory  DataStoreName=ADIAve_y_EMS_BrakePedalSignal  ShowAdditionalParam=off  StateMustResolveToSignalObject=on
  Data Store Memory29 : DataStoreMemory  DataStoreName=ADIAve_y_EMS_AccPedalFaultState  ShowAdditionalParam=off  StateMustResolveToSignalObject=on
  Data Store Memory3 : DataStoreMemory  DataStoreName=ADIAve_y_ESC_FRWhlSpdFaultSignal  ShowAdditionalParam=off  StateMustResolveToSignalObject=on
  Data Store Memory30 : DataStoreMemory  DataStoreName=ADIAve_y_Radar_State  ShowAdditionalParam=off  StateMustResolveToSignalObject=on
  Data Store Memory31 : DataStoreMemory  DataStoreName=ADIAve_y_Camera_State  ShowAdditionalParam=off  StateMustResolveToSignalObject=on
  Data Store Memory32 : DataStoreMemory  DataStoreName=ADIAve_y_SAS_SASFailureSt  ShowAdditionalParam=off  StateMustResolveToSignalObject=on
  Data Store Memory33 : DataStoreMemory  DataStoreName=ADIAve_y_BCM_LeftTurnSwSt  ShowAdditionalParam=off  StateMustResolveToSignalObject=on
  Data Store Memory34 : DataStoreMemory  DataStoreName=ADIAve_y_BCM_RightTurnSwSt  ShowAdditionalParam=off  StateMustResolveToSignalObject=on
  Data Store Memory35 : DataStoreMemory  DataStoreName=ADIAve_d_EMS_RealPTWhlTrq  ShowAdditionalParam=off  StateMustResolveToSignalObject=on
  Data Store Memory36 : DataStoreMemory  DataStoreName=ADIAve_g_EMS_MaxNoCtrlWhlTrqOst  ShowAdditionalParam=off  StateMustResolveToSignalObject=on
  Data Store Memory37 : DataStoreMemory  DataStoreName=ADIAve_g_EMS_MaxWhlTrq  ShowAdditionalParam=off  StateMustResolveToSignalObject=on
  Data Store Memory38 : DataStoreMemory  DataStoreName=ADIAve_g_EMS_MinNoCtrlWhlTrqOst  ShowAdditionalParam=off  StateMustResolveToSignalObject=on
  Data Store Memory39 : DataStoreMemory  DataStoreName=ADIAve_g_EMS_MinWhlTrq  ShowAdditionalParam=off  StateMustResolveToSignalObject=on
  Data Store Memory4 : DataStoreMemory  DataStoreName=ADIAve_y_ESC_RLWhlSpdFaultSignal  ShowAdditionalParam=off  StateMustResolveToSignalObject=on
  Data Store Memory40 : DataStoreMemory  DataStoreName=ADIAve_g_EMS_AccPdPositionRaw  ShowAdditionalParam=off  StateMustResolveToSignalObject=on
  Data Store Memory41 : DataStoreMemory  DataStoreName=ADIAve_g_EPS_SteerTrq  ShowAdditionalParam=off  StateMustResolveToSignalObject=on
  Data Store Memory42 : DataStoreMemory  DataStoreName=ADIAve_g_ESC_UnfltYawRate  ShowAdditionalParam=off  StateMustResolveToSignalObject=on
  Data Store Memory43 : DataStoreMemory  DataStoreName=ADIAve_y_Mp5_LSSMode  ShowAdditionalParam=off  StateMustResolveToSignalObject=on
  Data Store Memory44 : DataStoreMemory  DataStoreName=ADIAve_y_MP5_AEBSwitch  ShowAdditionalParam=off  StateMustResolveToSignalObject=on
  Data Store Memory45 : DataStoreMemory  DataStoreName=ADIAve_y_MP5_FCWSwitch  ShowAdditionalParam=off  StateMustResolveToSignalObject=on
  Data Store Memory46 : DataStoreMemory  DataStoreName=ADIAve_y_SCC_LeftSteerWhlSw  ShowAdditionalParam=off  StateMustResolveToSignalObject=on
  Data Store Memory47 : DataStoreMemory  DataStoreName=ADIAve_y_TCU_ActualGear  ShowAdditionalParam=off  StateMustResolveToSignalObject=on
  Data Store Memory48 : DataStoreMemory  DataStoreName=ADIAve_g_BCM_BattVolt  ShowAdditionalParam=off  StateMustResolveToSignalObject=on
  Data Store Memory49 : DataStoreMemory  DataStoreName=ADIAve_d_sen_sta_LF_radar  ShowAdditionalParam=off  StateMustResolveToSignalObject=on
  Data Store Memory5 : DataStoreMemory  DataStoreName=ADIAve_y_ESC_RRWhlSpdFaultSignal  ShowAdditionalParam=off  StateMustResolveToSignalObject=on
  Data Store Memory50 : DataStoreMemory  DataStoreName=ADIAve_d_sen_sta_RF_radar  ShowAdditionalParam=off  StateMustResolveToSignalObject=on
  Data Store Memory51 : DataStoreMemory  DataStoreName=ADIAve_d_sen_sta_LB_radar  ShowAdditionalParam=off  StateMustResolveToSignalObject=on
  Data Store Memory52 : DataStoreMemory  DataStoreName=ADIAve_d_sen_sta_RB_radar  ShowAdditionalParam=off  StateMustResolveToSignalObject=on
  Data Store Memory53 : DataStoreMemory  DataStoreName=ADIAve_g_ADAS_DecelerationSet  ShowAdditionalParam=off  StateMustResolveToSignalObject=on
  Data Store Memory54 : DataStoreMemory  DataStoreName=ADIAve_y_ADAS_ACCState  ShowAdditionalParam=off  StateMustResolveToSignalObject=on
  Data Store Memory55 : DataStoreMemory  DataStoreName=ADIAve_y_ADAS_AEBBrakingProg  ShowAdditionalParam=off  StateMustResolveToSignalObject=on
  Data Store Memory56 : DataStoreMemory  DataStoreName=ADIAve_y_ADAS_BrakeRequest  ShowAdditionalParam=off  StateMustResolveToSignalObject=on
  Data Store Memory57 : DataStoreMemory  DataStoreName=ADIAve_y_ADAS_DecelerationType  ShowAdditionalParam=off  StateMustResolveToSignalObject=on
  Data Store Memory58 : DataStoreMemory  DataStoreName=ADIAve_y_ADAS_DeclControlReq  ShowAdditionalParam=off  StateMustResolveToSignalObject=on
  Data Store Memory59 : DataStoreMemory  DataStoreName=ADIAve_y_ADAS_ESCDriveOff  ShowAdditionalParam=off  StateMustResolveToSignalObject=on
  Data Store Memory6 : DataStoreMemory  DataStoreName=ADIAve_y_EPS_SteerTrqSensorSt  ShowAdditionalParam=off  StateMustResolveToSignalObject=on
  Data Store Memory60 : DataStoreMemory  DataStoreName=ADIAve_y_ADAS_ESCHoldReq  ShowAdditionalParam=off  StateMustResolveToSignalObject=on
  Data Store Memory61 : DataStoreMemory  DataStoreName=ADIAve_y_ADAS_PrefillRequest  ShowAdditionalParam=off  StateMustResolveToSignalObject=on
  Data Store Memory62 : DataStoreMemory  DataStoreName=ADIAve_y_ADAS_TorqueActivReq  ShowAdditionalParam=off  StateMustResolveToSignalObject=on
  Data Store Memory63 : DataStoreMemory  DataStoreName=ADIAve_g_EMS_AccPedalPos  ShowAdditionalParam=off  StateMustResolveToSignalObject=on
  Data Store Memory64 : DataStoreMemory  DataStoreName=ADIAve_g_EMS_EngIndTrq  ShowAdditionalParam=off  StateMustResolveToSignalObject=on
  Data Store Memory65 : DataStoreMemory  DataStoreName=ADIAve_g_EPS_SteerAngle  ShowAdditionalParam=off  StateMustResolveToSignalObject=on
  Data Store Memory66 : DataStoreMemory  DataStoreName=ADIAve_g_ESC_BrkWhlCylPress  ShowAdditionalParam=off  StateMustResolveToSignalObject=on
  Data Store Memory67 : DataStoreMemory  DataStoreName=ADIAve_g_ESC_LateralAccel  ShowAdditionalParam=off  StateMustResolveToSignalObject=on
  Data Store Memory68 : DataStoreMemory  DataStoreName=ADIAve_g_ESC_LongitudinalAccel  ShowAdditionalParam=off  StateMustResolveToSignalObject=on
  Data Store Memory69 : DataStoreMemory  DataStoreName=ADIAve_g_ESC_VehSpd  ShowAdditionalParam=off  StateMustResolveToSignalObject=on
  Data Store Memory7 : DataStoreMemory  DataStoreName=ADIAve_y_TCU_ATFailure  ShowAdditionalParam=off  StateMustResolveToSignalObject=on
  Data Store Memory70 : DataStoreMemory  DataStoreName=ADIAve_g_ESC_YawRate  ShowAdditionalParam=off  StateMustResolveToSignalObject=on
  Data Store Memory71 : DataStoreMemory  DataStoreName=ADIAve_g_SAS_SteerAngle  ShowAdditionalParam=off  StateMustResolveToSignalObject=on
  Data Store Memory72 : DataStoreMemory  DataStoreName=ADIAve_g_SAS_SteerRotSpd  ShowAdditionalParam=off  StateMustResolveToSignalObject=on
  Data Store Memory73 : DataStoreMemory  DataStoreName=ADIAve_y_ESC_BrkReleaseFailsafe  ShowAdditionalParam=off  StateMustResolveToSignalObject=on
  Data Store Memory74 : DataStoreMemory  DataStoreName=ADIAve_y_ESC_DynSlope  ShowAdditionalParam=off  StateMustResolveToSignalObject=on
  Data Store Memory75 : DataStoreMemory  DataStoreName=ADIAve_y_ESC_DynSlopeAccuracy  ShowAdditionalParam=off  StateMustResolveToSignalObject=on
  Data Store Memory76 : DataStoreMemory  DataStoreName=ADIAve_y_ESC_StaticSlope  ShowAdditionalParam=off  StateMustResolveToSignalObject=on
  Data Store Memory77 : DataStoreMemory  DataStoreName=ADIAve_y_ESC_VehHoldState  ShowAdditionalParam=off  StateMustResolveToSignalObject=on
  Data Store Memory78 : DataStoreMemory  DataStoreName=ADIAve_y_SAS_TrimState  ShowAdditionalParam=off  StateMustResolveToSignalObject=on
  Data Store Memory79 : DataStoreMemory  DataStoreName=ADIAve_e_Node_ACU_Validity  InitialValue=SPARte_e_Validity.SPARce_e_Valid  ShowAdditionalParam=off  StateMustResolveToSignalObject=on
  Data Store Memory8 : DataStoreMemory  DataStoreName=ADIAve_y_ESC_ABSValidity  ShowAdditionalParam=off  StateMustResolveToSignalObject=on
  Data Store Memory80 : DataStoreMemory  DataStoreName=ADIAve_e_Node_EPS_Validity  InitialValue=SPARte_e_Validity.SPARce_e_Valid  ShowAdditionalParam=off  StateMustResolveToSignalObject=on
  Data Store Memory81 : DataStoreMemory  DataStoreName=ADIAve_e_Node_ESC_Validity  InitialValue=SPARte_e_Validity.SPARce_e_Valid  ShowAdditionalParam=off  StateMustResolveToSignalObject=on
  Data Store Memory82 : DataStoreMemory  DataStoreName=ADIAve_e_Node_IBCM_Validity  InitialValue=SPARte_e_Validity.SPARce_e_Valid  ShowAdditionalParam=off  StateMustResolveToSignalObject=on
  Data Store Memory83 : DataStoreMemory  DataStoreName=ADIAve_e_Node_SAS_Validity  InitialValue=SPARte_e_Validity.SPARce_e_Valid  ShowAdditionalParam=off  StateMustResolveToSignalObject=on
  Data Store Memory84 : DataStoreMemory  DataStoreName=ADIAve_e_Node_EMS_Validity  InitialValue=SPARte_e_Validity.SPARce_e_Valid  ShowAdditionalParam=off  StateMustResolveToSignalObject=on
  Data Store Memory85 : DataStoreMemory  DataStoreName=ADIAve_e_Node_IC_Validity  InitialValue=SPARte_e_Validity.SPARce_e_Valid  ShowAdditionalParam=off  StateMustResolveToSignalObject=on
  Data Store Memory86 : DataStoreMemory  DataStoreName=ADIAve_e_Node_TBOX_Validity  InitialValue=SPARte_e_Validity.SPARce_e_Valid  ShowAdditionalParam=off  StateMustResolveToSignalObject=on
  Data Store Memory87 : DataStoreMemory  DataStoreName=ADIAve_e_Node_MP5_Validity  InitialValue=SPARte_e_Validity.SPARce_e_Valid  ShowAdditionalParam=off  StateMustResolveToSignalObject=on
  Data Store Memory88 : DataStoreMemory  DataStoreName=ADIAve_e_Node_TCU_Validity  InitialValue=SPARte_e_Validity.SPARce_e_Valid  ShowAdditionalParam=off  StateMustResolveToSignalObject=on
  Data Store Memory89 : DataStoreMemory  DataStoreName=ADIAve_e_Node_EPB_Validity  InitialValue=SPARte_e_Validity.SPARce_e_Valid  ShowAdditionalParam=off  StateMustResolveToSignalObject=on
  Data Store Memory9 : DataStoreMemory  DataStoreName=ADIAve_y_ESC_ESCValidity  ShowAdditionalParam=off  StateMustResolveToSignalObject=on
  Data Store Memory90 : DataStoreMemory  DataStoreName=ADIAve_b_DTCOperationCycle  ShowAdditionalParam=off  StateMustResolveToSignalObject=on
  Data Store Memory91 : DataStoreMemory  DataStoreName=ADIA_DTC_EMS_14B_InvOorRealWhlTrq  ShowAdditionalParam=off  StateMustResolveToSignalObject=on
  Data Store Memory92 : DataStoreMemory  DataStoreName=ADIA_DTC_EMS_17E_InvOorMaxNotContrlWhlTrq  ShowAdditionalParam=off  StateMustResolveToSignalObject=on
  Data Store Memory93 : DataStoreMemory  DataStoreName=ADIA_DTC_EMS_17E_InvOorMaxTrqWhl  ShowAdditionalParam=off  StateMustResolveToSignalObject=on
  Data Store Memory94 : DataStoreMemory  DataStoreName=ADIA_DTC_EMS_17E_InvOorMinTrqWhl  ShowAdditionalParam=off  StateMustResolveToSignalObject=on
  Data Store Memory95 : DataStoreMemory  DataStoreName=ADIA_DTC_EMS_17E_InvOorMinNotContrlWhlTrq  ShowAdditionalParam=off  StateMustResolveToSignalObject=on
  Data Store Memory96 : DataStoreMemory  DataStoreName=ADIA_DTC_BatteryOutOfRange  ShowAdditionalParam=off  StateMustResolveToSignalObject=on
  Data Store Memory97 : DataStoreMemory  DataStoreName=ADIA_Inner_FRadar_FaultState  ShowAdditionalParam=off  StateMustResolveToSignalObject=on
  Data Store Memory98 : DataStoreMemory  DataStoreName=ob_ADIAve_g_ASWFaultStatus_ini  ShowAdditionalParam=off  StateMustResolveToSignalObject=on
  Data Store Memory99 : DataStoreMemory  DataStoreName=ob_ADIAve_d_FuncFaultStatus_ini  ShowAdditionalParam=off  StateMustResolveToSignalObject=on
  Data Store Read : DataStoreRead  DataStoreName=ADIA_DTC_EMS_17E_InvOorMinNotContrlWhlTrq
  Data Type Conversion : DataTypeConversion  OutDataTypeStr=uint16
  Data Type Conversion1 : DataTypeConversion
  Data Type Conversion2 : DataTypeConversion
  Data Type Conversion3 : DataTypeConversion  OutDataTypeStr=single
  Data Type Conversion4 : DataTypeConversion  OutDataTypeStr=boolean
  Diagnostics_Processing : Subsystem
  Get_Public_Data : Subsystem
  ModelVersion : Constant  Value=01001  OutDataTypeStr=uint16  SampleTime=-1
  Output_Processing : Subsystem
  Processing : Stateflow chart  TreatAsAtomicUnit=on
  Terminator : Terminator
  Terminator1 : Terminator
  Terminator2 : Terminator
  ADIAve_g_ASWFaultStatus : Outport
  ADIAve_g_BSWFaultStatus : Outport  Port=2
  ADIAve_d_FuncFaultStatus : Outport  Port=3
  wires:
  Processing/3(GetData()) -> [GetData]
  Processing/4(Process()) -> [Process]
  Processing/5(Output()) -> [Output]
  SWINve_y_ESC_VehSpdValidFlag/1 -> Get_Public_Data/1(SWINve_y_ESC_VehSpdValidFlag)
  SWINve_y_ESC_FLWHeelSpdFaultSignal/1 -> Get_Public_Data/2(SWINve_y_ESC_FLWHeelSpdFaultSignal)
  SWINve_y_ESC_FRWHeelSpdFaultSignal/1 -> Get_Public_Data/3(SWINve_y_ESC_FRWHeelSpdFaultSignal)
  SWINve_y_ESC_RLWHeelSpdFaultSignal/1 -> Get_Public_Data/4(SWINve_y_ESC_RLWHeelSpdFaultSignal)
  SWINve_y_ESC_RRWHeelSpdFaultSignal/1 -> Get_Public_Data/5(SWINve_y_ESC_RRWHeelSpdFaultSignal)
  SWINve_y_EPS_SteerintTorqueSensorSt/1 -> Get_Public_Data/6(SWINve_y_EPS_SteerintTorqueSensorSt)
  SWINve_y_TCU_ATFailure/1 -> Get_Public_Data/7(SWINve_y_TCU_ATFailure)
  SWINve_y_ESC_ABSValidity/1 -> Get_Public_Data/8(SWINve_y_ESC_ABSValidity)
  SWINve_y_ESC_ESCValidity/1 -> Get_Public_Data/9(SWINve_y_ESC_ESCValidity)
  SWINve_y_EMS_ACCResponseStatus/1 -> Get_Public_Data/10(SWINve_y_EMS_ACCResponseStatus)
  SWINve_y_BCM_CHMSLStaus/1 -> Get_Public_Data/11(SWINve_y_BCM_CHMSLStaus)
  SWINve_y_BCM_BrakeLampStaus/1 -> Get_Public_Data/12(SWINve_y_BCM_BrakeLampStaus)
  SWINve_y_EMS_EngRunningStatus/1 -> Get_Public_Data/13(SWINve_y_EMS_EngRunningStatus)
  SWINve_y_EPS_SteeringAngle_Flag/1 -> Get_Public_Data/14(SWINve_y_EPS_SteeringAngle_Flag)
  SWINve_y_EPS_LKAState/1 -> Get_Public_Data/15(SWINve_y_EPS_LKAState)
  SWINve_y_EPS_ESAState/1 -> Get_Public_Data/16(SWINve_y_EPS_ESAState)
  SWINve_y_ESC_TCSCtlActive/1 -> Get_Public_Data/17(SWINve_y_ESC_TCSCtlActive)
  SWINve_y_ESC_TCSErrorStatus/1 -> Get_Public_Data/18(SWINve_y_ESC_TCSErrorStatus)
  SWINve_y_ESC_VehicleStandstill/1 -> Get_Public_Data/19(SWINve_y_ESC_VehicleStandstill)
  SWINve_y_ESC_YawrateValidity/1 -> Get_Public_Data/20(SWINve_y_ESC_YawrateValidity)
  SWINve_y_ESC_LateralAccelarationValidity/1 -> Get_Public_Data/21(SWINve_y_ESC_LateralAccelarationValidity)
  SWINve_y_ESC_LongitudinalAccelervalidity/1 -> Get_Public_Data/22(SWINve_y_ESC_LongitudinalAccelervalidity)
  SWINve_y_ESC_VehDrivingDirection/1 -> Get_Public_Data/23(SWINve_y_ESC_VehDrivingDirection)
  SWINve_y_ESC_EPBSwitchStaticsValidity/1 -> Get_Public_Data/24(SWINve_y_ESC_EPBSwitchStaticsValidity)
  SWINve_y_ESC_EPBErrorStatus/1 -> Get_Public_Data/25(SWINve_y_ESC_EPBErrorStatus)
  SWINve_y_Mp5_ISASwitch/1 -> Get_Public_Data/26(SWINve_y_Mp5_ISASwitch)
  SWINve_y_Mp5_ISAMode/1 -> Get_Public_Data/27(SWINve_y_Mp5_ISAMode)
  SWINve_y_EMS_BrakePedalSignal/1 -> Get_Public_Data/28(SWINve_y_EMS_BrakePedalSignal)
  SWINve_y_EMS_AccPedalFaultBit/1 -> Get_Public_Data/29(SWINve_y_EMS_AccPedalFaultBit)
  SDFAve_y_Radar_State/1 -> Get_Public_Data/30(SDFAve_y_Radar_State)
  SDFAve_y_OperatingStatus/1 -> Get_Public_Data/31(SDFAve_y_OperatingStatus)
  SWINve_y_SAS_SASFailureSts/1 -> Get_Public_Data/32(SWINve_y_SAS_SASFailureSts)
  SWINve_y_BCM_LeftTurnSwitchSt/1 -> Get_Public_Data/33(SWINve_y_BCM_LeftTurnSwitchSt)
  SWINve_y_BCM_RightTurnSwitchSt/1 -> Get_Public_Data/34(SWINve_y_BCM_RightTurnSwitchSt)
  SWINve_d_EMS_RealizedPowertrainWheelTorq/1 -> Get_Public_Data/35(SWINve_d_EMS_RealizedPowertrainWheelTorq)
  SWINve_g_EMS_NotControlableMaxPowertra/1 -> Get_Public_Data/36(SWINve_g_EMS_NotControlableMaxPowertra)
  SWINve_g_EMS_MaxPowertrainWheelTorque/1 -> Get_Public_Data/37(SWINve_g_EMS_MaxPowertrainWheelTorque)
  SWINve_g_EMS_NotControlableMinPowertra/1 -> Get_Public_Data/38(SWINve_g_EMS_NotControlableMinPowertra)
  SWINve_g_EMS_MinPowertrainWheelTorque/1 -> Get_Public_Data/39(SWINve_g_EMS_MinPowertrainWheelTorque)
  SWINve_g_EMS_AccPedalPositionRaw/1 -> Get_Public_Data/40(SWINve_g_EMS_AccPedalPositionRaw)
  SWINve_g_EPS_SteeringTorqueValue/1 -> Get_Public_Data/41(SWINve_g_EPS_SteeringTorqueValue)
  SWINve_g_ESC_UnfilteredYawRate/1 -> Get_Public_Data/42(SWINve_g_ESC_UnfilteredYawRate)
  SWINve_y_Mp5_LSSMode/1 -> Get_Public_Data/43(SWINve_y_Mp5_LSSMode)
  SWINve_y_MP5_AEBSwitch/1 -> Get_Public_Data/44(SWINve_y_MP5_AEBSwitch)
  SWINve_y_MP5_FCWSwitch/1 -> Get_Public_Data/45(SWINve_y_MP5_FCWSwitch)
  SWINve_y_SCC_LeftSteeringWheelSwitchSig/1 -> Get_Public_Data/46(SWINve_y_SCC_LeftSteeringWheelSwitchSig)
  SWINve_y_TCU_ActialGear/1 -> Get_Public_Data/47(SWINve_y_TCU_ActialGear)
  SWINve_g_BCM_BattVolt/1 -> Get_Public_Data/48(SWINve_g_BCM_BattVolt)
  CANEve_e_Node_ACU_Validity/1 -> Get_Public_Data/49(CANEve_e_Node_ACU_Validity)  "ob_ADIAve_e_Node_ACU_Validity"
  CANEve_e_Node_EPS_Validity/1 -> Get_Public_Data/50(CANEve_e_Node_EPS_Validity)  "ob_ADIAve_e_Node_EPS_Validity"
  CANEve_e_Node_ESC_Validity/1 -> Get_Public_Data/51(CANEve_e_Node_ESC_Validity)  "ob_ADIAve_e_Node_ESC_Validity"
  CANEve_e_Node_IBCM_Validity/1 -> Get_Public_Data/52(CANEve_e_Node_IBCM_Validity)  "ob_ADIAve_e_Node_IBCM_Validity"
  CANEve_e_Node_SAS_Validity/1 -> Get_Public_Data/53(CANEve_e_Node_SAS_Validity)  "ob_ADIAve_e_Node_SAS_Validity"
  CANEve_e_Node_EMS_Validity/1 -> Get_Public_Data/54(CANEve_e_Node_EMS_Validity)  "ob_ADIAve_e_Node_EMS_Validity"
  CANEve_e_Node_IC_Validity/1 -> Get_Public_Data/55(CANEve_e_Node_IC_Validity)  "ob_ADIAve_e_Node_IC_Validity"
  CANEve_e_Node_TBOX_Validity/1 -> Get_Public_Data/56(CANEve_e_Node_TBOX_Validity)  "ob_ADIAve_e_Node_TBOX_Validity"
  CANEve_e_Node_MP5_Validity/1 -> Get_Public_Data/57(CANEve_e_Node_MP5_Validity)  "ob_ADIAve_e_Node_MP5_Validity"
  CANEve_e_Node_TCU_Validity/1 -> Get_Public_Data/58(CANEve_e_Node_TCU_Validity)  "ob_ADIAve_e_Node_TCU_Validity"
  CANEve_e_Node_EPB_Validity/1 -> Get_Public_Data/59(CANEve_e_Node_EPB_Validity)  "ob_ADIAve_e_Node_EPB_Validity"
  SDFAve_d_sen_sta_LF_radar/1 -> Get_Public_Data/60(SDFAve_d_sen_sta_LF_radar)
  SDFAve_d_sen_sta_RF_radar/1 -> Get_Public_Data/61(SDFAve_d_sen_sta_RF_radar)
  SDFAve_d_sen_sta_LB_radar/1 -> Get_Public_Data/62(SDFAve_d_sen_sta_LB_radar)
  SDFAve_d_sen_sta_RB_radar/1 -> Get_Public_Data/63(SDFAve_d_sen_sta_RB_radar)
  AFDMve_b_DTCOperationCycle/1 -> Get_Public_Data/64(AFDMve_b_DTCOperationCycle)
  [GetData] -> Get_Public_Data/Trigger
  Output_Processing/1(ADIAve_g_ASWFaultStatus) -> ADIAve_g_ASWFaultStatus/1
  Output_Processing/2(ADIAve_g_BSWFaultStatus) -> ADIAve_g_BSWFaultStatus/1
  Output_Processing/3(ADIAve_d_FuncFaultStatus) -> ADIAve_d_FuncFaultStatus/1
  OMAPve_g_ADAS_ACCTorqueReq/1 -> Get_Public_Data/65(OMAPve_g_ADAS_ACCTorqueReq)
  OMAPve_g_ADAS_DecelerationSet/1 -> Get_Public_Data/66(OMAPve_g_ADAS_DecelerationSet)
  OMAPve_y_ADAS_ACCState/1 -> Get_Public_Data/67(OMAPve_y_ADAS_ACCState)
  OMAPve_y_ADAS_AEBBrakingProg/1 -> Get_Public_Data/68(OMAPve_y_ADAS_AEBBrakingProg)
  OMAPve_y_ADAS_BrakeRequest/1 -> Get_Public_Data/69(OMAPve_y_ADAS_BrakeRequest)
  OMAPve_y_ADAS_DecelerationType/1 -> Get_Public_Data/70(OMAPve_y_ADAS_DecelerationType)
  OMAPve_y_ADAS_DeclControlReq/1 -> Get_Public_Data/71(OMAPve_y_ADAS_DeclControlReq)
  OMAPve_y_ADAS_PrefillRequest/1 -> Get_Public_Data/74(OMAPve_y_ADAS_PrefillRequest)
  OMAPve_y_ADAS_ESCDriveOff/1 -> Get_Public_Data/72(OMAPve_y_ADAS_ESCDriveOff)
  OMAPve_y_ADAS_TorqueActivReq/1 -> Get_Public_Data/75(OMAPve_y_ADAS_TorqueActivReq)
  OMAPve_y_ADAS_ESCHoldReq/1 -> Get_Public_Data/73(OMAPve_y_ADAS_ESCHoldReq)
  SWINve_g_EMS_AccPedalPos/1 -> Get_Public_Data/76(SWINve_g_EMS_AccPedalPos)
  SWINve_g_ESC_BrakeWheelCylinderPressure/1 -> Get_Public_Data/79(SWINve_g_ESC_BrakeWheelCylinderPressure)
  SWINve_g_EMS_EngActualIndTorque/1 -> Get_Public_Data/77(SWINve_g_EMS_EngActualIndTorque)
  SWINve_g_ESC_LateralAccelaration/1 -> Get_Public_Data/80(SWINve_g_ESC_LateralAccelaration)
  SWINve_g_ESC_LongitudinalAcceleration/1 -> Get_Public_Data/81(SWINve_g_ESC_LongitudinalAcceleration)
  SWINve_g_EPS_SteeringAngle/1 -> Get_Public_Data/78(SWINve_g_EPS_SteeringAngle)
  SWINve_g_ESC_VeSpd/1 -> Get_Public_Data/82(SWINve_g_ESC_VeSpd)
  SWINve_g_ESC_YawRate/1 -> Get_Public_Data/83(SWINve_g_ESC_YawRate)
  SWINve_g_SAS_SteeringAngle/1 -> Get_Public_Data/84(SWINve_g_SAS_SteeringAngle)
  SWINve_g_SAS_SteeringRotSpd/1 -> Get_Public_Data/85(SWINve_g_SAS_SteeringRotSpd)
  SWINve_y_ESC_DynamicSlopeAccuracy/1 -> Get_Public_Data/88(SWINve_y_ESC_DynamicSlopeAccuracy)
  SWINve_y_ESC_BrakeReleasedFailsafe/1 -> Get_Public_Data/86(SWINve_y_ESC_BrakeReleasedFailsafe)
  SWINve_y_ESC_DynamicSlope/1 -> Get_Public_Data/87(SWINve_y_ESC_DynamicSlope)
  SWINve_y_ESC_Static_slope/1 -> Get_Public_Data/89(SWINve_y_ESC_Static_slope)
  SWINve_y_ESC_VehicleHoldStatus/1 -> Get_Public_Data/90(SWINve_y_ESC_VehicleHoldStatus)
  SWINve_y_SAS_TrimmingStatus/1 -> Get_Public_Data/91(SWINve_y_SAS_TrimmingStatus)
  [Process] -> Diagnostics_Processing/Trigger
  [Output] -> Output_Processing/Trigger
  ModelVersion/1 -> Data Type Conversion/1
  Data Type Conversion/1 -> Terminator/1  "ob_ADIA_ModelVersion"
  Constant10/1 -> Data Type Conversion2/1
  Constant/1 -> Data Type Conversion1/1
  Data Type Conversion1/1 -> Processing/2(DelayTime)
  Data Type Conversion2/1 -> Processing/1(dT)
  Processing/1(Timer) -> Data Type Conversion3/1
  Processing/2(Diag_Trigger) -> Data Type Conversion4/1
  Data Type Conversion3/1 -> Terminator1/1  "ob_ADIA_Diag_DelayTimer"
  Data Type Conversion4/1 -> Terminator2/1  "ob_ADIA_Diag_Trigger"
